simulink model "xue_flatness"  (R2017b)
settings: Solver=VariableStepAuto  StartTime=0.0  StopTime=58  RelTol=1e-9
libraries: simulink x1
(part 3 of 3)

== matlab function xue_flatness/Motor Mixing Algorithm ==
  data: parameters output; u output; parameters input size=8; u input size=4; rotor_speed_square output size=4
function [parameters,u,rotor_speed_square]=fcn(parameters,u)
l=parameters(6) ; 
k=parameters(7) ;
c=parameters(8) ;
rotor_speed_square=[1 0 -1  1;
                    1 1  0 -1;
                    1 0  1  1;
                    1 -1 0 -1]* [1/(4*k) 0         0         0;
                                0        1/(2*l*k) 0         0;
                                0        0         1/(2*l*k) 0;
                                0        0         0         1/(4*c)]*u ;
end
%% Motor dynamics
% rotor_speed=in(9:12)
% rotor_speed_square=rotor_speed.^2
%f_taux_tauy_tauz=[k 0   0   0;
%                  0 k*l 0   0;
%                  0 0   k*l 0;
%                  0 0   0   c]*[1  1 1  1;
%                                0  1 0 -1;
%                               -1  0 1  0;
%                                1 -1 1 -1]*rotor_speed_square

== matlab function xue_flatness/Rigid Body Dynamics ==
  data: parameters input size=8; x_dot output size=12; u input size=4; x input size=12
function x_dot=fcn(parameters,u,x)
%% allocate inputs
m=parameters(1);
g=parameters(2);
M=diag([parameters(3) parameters(4) parameters(5)]);
f=u(1);
taub=u(2:4);
pn=x(1:3);
vn=x(4:6);
eta=x(7:9);
omegab=x(10:12);
%% define matrix Rbn , Lbn and Omega
phi=eta(1);
theta=eta(2);
psi=eta(3);
Rbn=[cos(theta)*cos(psi) sin(phi)*sin(theta)*cos(psi)-cos(phi)*sin(psi) cos(phi)*sin(theta)*cos(psi)+sin(phi)*sin(psi);
     cos(theta)*sin(psi) sin(phi)*sin(theta)*sin(psi)+cos(phi)*cos(psi) cos(phi)*sin(theta)*sin(psi)-sin(phi)*cos(psi);
     -sin(theta)         sin(phi)*cos(theta)                            cos(phi)*cos(theta)                           ];
Lbn=[1 sin(phi)*tan(theta) cos(phi)*tan(theta);
     0 cos(phi)            -sin(phi);
     0 sin(phi)/cos(theta) cos(phi)/cos(theta)];

%% nonlinear model: shown on the handout
pn_dot=vn;
vn_dot=1/m*Rbn*[0 0 f]'-[0 0 g]'; % -1/m*[Ax 0 0;0 Ay 0;0 0 Az]*pn_dot;    % pay attention to whether I need Ax, Ay, Az
eta_dot=Lbn*omegab;
omegab_dot=M\(taub-cross(omegab,M*omegab));
%% output x_dot
x_dot=[pn_dot;
       vn_dot;
       eta_dot;
       omegab_dot];
end
